simulink model "mpcsimulink"  (R2020a)
settings: Solver=VariableStepAuto  StartTime=0.0  StopTime=60  RelTol=1e-3
values from neighbouring files (symbols this model uses):
  d = 1    [INIT.m]    (also in INITKF.m; INITexp.m; INITnonmpc.m; pendcont.m)
  D = 0    [INIT.m]    (also in INITexp.m; pendcont.m = m*L*L*(M+m*(1-Cy^2)))
  g = -10    [INIT.m]    (also in INITKF.m; INITexp.m = -9.8; INITnonmpc.m = -9.8; pendcont.m = -9.8)
  K = lqr(A,B,Q,R)    [INIT.m]    (also in INITKF.m; INITexp.m; INITnonmpc.m)
  L = 2    [INIT.m]    (also in INITKF.m; INITexp.m = 0.07; INITnonmpc.m = 0.06; pendcont.m = 0.06)
  M = 5    [INIT.m]    (also in INITKF.m; INITexp.m = 0.32; INITnonmpc.m = 0.08; pendcont.m = 0.08)
  m = 1    [INIT.m]    (also in INITKF.m; INITexp.m = 0.25; INITnonmpc.m = 0.01; pendcont.m = 0.01)
  Ts = 0.1    [INITnonmpc.m]
libraries: mpclib x1
settings Model: Creator=Prodigio  LastModifiedBy=Prodigio

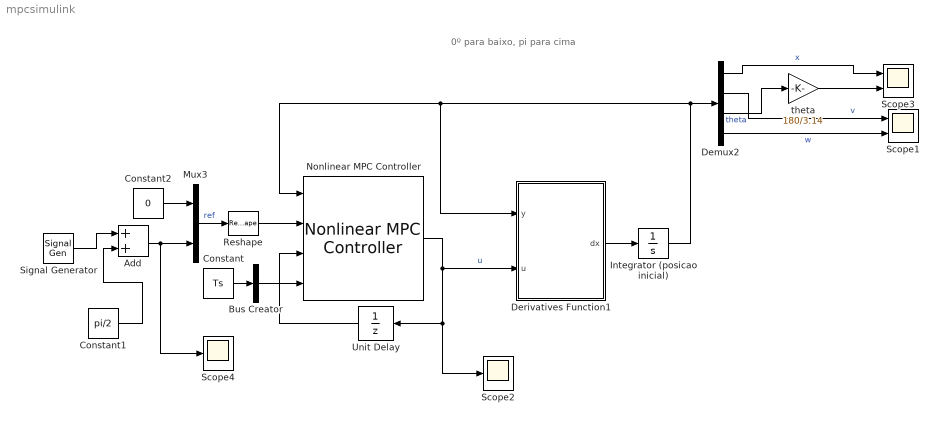
== system mpcsimulink ==
  note: 0º para baixo, pi para cima
  Add : Sum
  Bus Creator : BusCreator  Inputs=1  OutDataTypeStr=Bus: BusNMPC  NonVirtualBus=on
      settings: InheritFromInputs=off
  Constant : Constant  Value=Ts
  Constant1 : Constant  Value=pi/2
  Constant2 : Constant  Value=0
  Demux2 : Demux
  Derivatives Function1 : MATLAB Function  TreatAsAtomicUnit=on
  Integrator (posicao inicial) : Integrator  InitialCondition=[0;0;0;0]
  Mux3 : Mux  Inputs=2
  Nonlinear MPC Controller : mpclib/Nonlinear MPC Controller  SCDEnableBlockLinearizationSpecification=on  nlmpcobj=nlobj  UseObjectTs=on  UseMEX=off  md_enabled=off  mvtarget_enabled=off  param_enabled=on  cost_enabled=off  mvseq_enabled=off  stateseq_enabled=off  ovseq_enabled=off  slack_enabled=off  status_enabled=off  ov_min=off  ov_max=off  mv_min=off  mv_max=off  mvrate_min=off  mvrate_max=off  state_min=off  state_max=off  ov_weight=off  mv_weight=off  mvrate_weight=off  ecr_weight=off  nlp_initialize=off
  Reshape : Reshape  OutputDimensionality=Row vector (2-D)
  Scope1 : Scope  NumInputPorts=2
  Scope2 : Scope
  Scope3 : Scope  NumInputPorts=2
  Scope4 : Scope
  Signal Generator : SignalGenerator  WaveForm=square  Amplitude=pi/2  Frequency=0.05
  Unit Delay : UnitDelay  SampleTime=-1  HasFrameUpgradeWarning=on
  theta : Gain  Gain=180/3.14
  wires:
  Integrator (posicao inicial)/1 -> Derivatives Function1/1(y), Nonlinear MPC Controller/1, Demux2/1
  Constant1/1 -> Add/2
  Signal Generator/1 -> Add/1
  Reshape/1 -> Nonlinear MPC Controller/2
  Unit Delay/1 -> Nonlinear MPC Controller/3
  Demux2/3 -> theta/1  "theta"
  Constant/1 -> Bus Creator/1
  Nonlinear MPC Controller/1 -> Unit Delay/1, Scope2/1, Derivatives Function1/2(u)  "u"
  theta/1 -> Scope3/2
  Mux3/1 -> Reshape/1  "ref"
  Derivatives Function1/1(dx) -> Integrator (posicao inicial)/1
  Demux2/1 -> Scope3/1  "x"
  Demux2/4 -> Scope1/2  "w"
  Demux2/2 -> Scope1/1  "v"
  Bus Creator/1 -> Nonlinear MPC Controller/4
  Constant2/1 -> Mux3/1
  Add/1 -> Mux3/2, Scope4/1

== matlab function mpcsimulink/Derivatives Function1 ==
  settings: updateMethod=CONTINUOUS
  data: y input; dx output; m parameter; M parameter; L parameter; g parameter; d parameter; K parameter; u input
function dx = derivativesexp(y,m, M, L, g, d, K,u)
% y = [x , ^x, o , ^o] states , y=xdot
% M massa do carro, m massa do pendulo, L tamanho do fio
% d fricÃ§ao, g grav no pendulo

dx=0*y;
dx=pendcont(y,u);

% Sy = sin(y(3));
% Cy = cos(y(3));
% D = m*L*L*(M+m*(1-Cy^2));

% setpoints
% newx = [2; 0; pi; 0];
% newx = [0; 0; 0; 0];
% 
% % if(t>12)
% %     newx = [-1; 0; pi; 0]; 
% % end 
% 
% % open loop (no control)
% % if(t>29)
% %   u = 0;
% % else
%                                             % && u ~= 0
% if (( y(3) > (pi-pi/5) ) && ( y(3) < (pi+pi/5)) || ...
%    ( y(3) > (-pi-pi/5) ) && ( y(3) < (-pi+pi/5)) )  
%     u = K * ([0;0;pi;0] - [y(1);y(2);y(3);y(4)]); % lqr control u = k*(newx-x)
% else
%     % energy based swing-up control % 1996 furata and astrom eq.6
%     % E=2/3*m2*l^2*x(4)^2 - m2*g*l*(cos(x(3))-1);
%     % u=0.2*m1*E*x(4)*cos(x(3));
% %         k=1;
% %         Ed= -m*g*L*cos(pi);
% %         E= m*L^2*y(4) - m*g*L*cos(y(3));
% %         u=k*y(4)*(E-Ed);
%      E= m*g*L*(cos(y(3)));
%      u=0.8*M*E*y(4)*(cos(y(3))); %velocidade com que ganha balanço, 0.8 ou o primeiro valor serve como tunning
% %     end
% end



%derivadas 

% dx=pendcont(y,u)

% -m*m*l*l*g*Sy*Sy
% m*l*l*m*l*y(4)^2*Sy
% %-m*l*l*d*y(2)
% %m*l*l*u
% 
% (m+M)*m*g*l*Sy
% m*l*Cy*m*l*y(4)^2*Sy
% %-m*l*Cy*d*y(2)
% %m*l*Cy*u
